simulink model "ACC_CC_model_best_2017aV1"  (Simulink 9.0)
settings: Solver=FixedStepAuto  StartTime=0.0  StopTime=1000  RelTol=1e-3
InitFcn:
  | step=0.001;%时间步长
  | run par.m
values from neighbouring files (symbols this model uses):
  ax_1 = Pop(i,1)    [IGPSO.m]
  ax_2 = Pop(i,2)    [IGPSO.m]
  ess_init_soc = 0.9    [IGPSO.m]
  ess_max_ah_cap = 5    [IGPSO.m]
  ess_r_chg = [0.001393 0.001393 0.001393 0.001393 0.001256 0.001172 0.001099 0.001074 0.001058 0.001066 0.0011 0.001161 0.001244 0.001327 0.001327]*3/5*32    [IGPSO.m]
  ess_r_dis = [0.004178 0.004178 0.004178 0.004178 0.003769 0.003517 0.003296 0.003222 0.003173 0.003197 0.0033 0.003483 0.003732 0.00398 0.00398]*3/5*32    [IGPSO.m]
  ess_soc = [0 0.2 0.25 0.3 0.35 0.4 0.45 0.5 0.55 0.6 0.65 0.7 0.75 0.8 1]    [IGPSO.m]
  ess_voc = [3.124 3.36 3.42 3.479 3.501 3.524 3.547 3.569 3.593 3.616 3.65 3.684 3.72 3.756 3.9]*3*32    [IGPSO.m]
  mc_eff_map = [0.43,0.49,0.58,0.66,0.73,0.70,0.73,0.66,0.58,0.49,0.43 ... (first row only)    [IGPSO.m]
  mc_map_spd = [0;1000;2000;3000;3500;4000;5000;6000;6500;7000;8000]*(2*pi)/60    [IGPSO.m]
  mc_map_trq = motorMAP(1,2:end)    [IGPSO.m]
  mc_max_trq = [142.2;148.6;146.5;92.4;83.9;71.1;56.9;48.4;43.4;37.7;35.6]    [IGPSO.m]
  v_base = 30    [IGPSO.m]
libraries: simulink x2, Solver_SF x1
(part 1 of 2)
settings Model: Creator=Administrator  LastModifiedBy=61602
settings DataIOCC: SaveFormat=Dataset
settings OptimizationCC: LifeSpan=auto
settings DebuggingCC: UnderspecifiedInitializationDetection=Simplified  MergeDetectMultiDrivingBlocksExec=error  SFUnexpectedBacktrackingDiag=error  SFNoUnconditionalDefaultTransitionDiag=error  SFExecutionAtInitializationDiag=warning
settings HardwareCC: ProdBitPerPointer=64  ProdBitPerSizeT=64  ProdBitPerPtrDiffT=64  ProdLargestAtomicFloat=Float  ProdIntDivRoundTo=Zero  ProdEndianess=LittleEndian  ProdWordSize=64  ProdHWDeviceType=Intel->x86-64 (Windows64)
settings ModelReferenceCC: PropagateSignalLabelsOutOfModel=on
settings GRTTargetCC: TargetLangStandard=C99 (ISO)
settings ConfigComp: CovMetricSettings=dwe  CovHtmlReporting=off  CovSaveCumulativeToWorkspaceVar=off  CovSaveSingleToWorkspaceVar=off  CovExternalEMLEnable=on

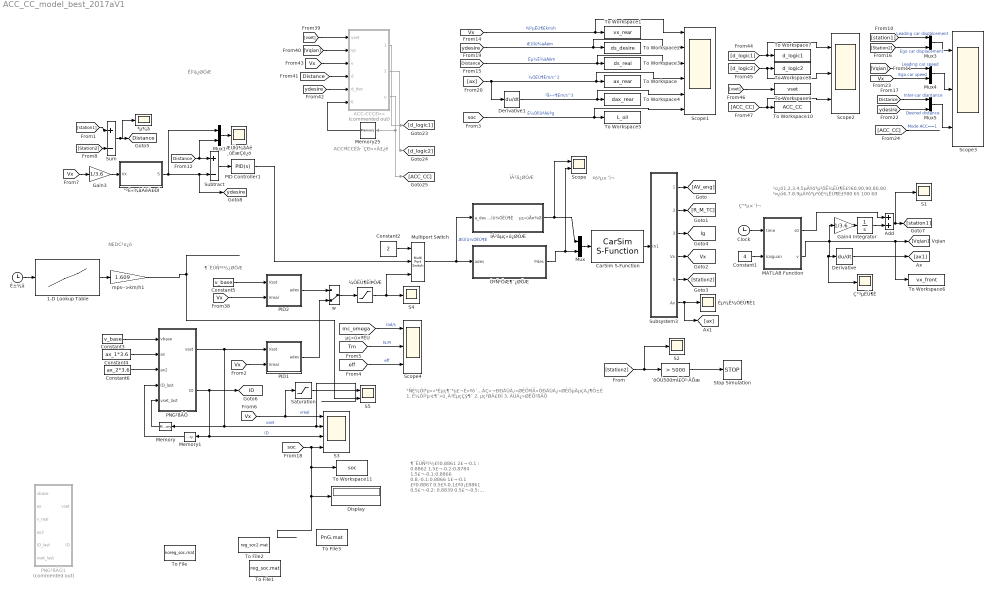
== system ACC_CC_model_best_2017aV1 ==
  note: NEDC工况
  note: 把燃油车换成电动车，然后搭建电池模型，能量回收策略模型png滑行最优加速度用粒子群或者遗传算法优化去做，最后对比考虑滑行能量回收和没有能量回收的电量对比
      | 1. 燃油车发动机改成电驱动
      | 2. 电池模型
      | 3. 能量回收策略
  note: ACC和CC算法切换模块
  note: 工况1,2,3,4,5的后车初始速度：60,90,90,80,80
      | 工况6.7.8.9的后车初始速度：80   65 100 60
  note: 下层控制
  note: 定速巡航控制
  note: 前车状态
  note: 后车状态
  note: 上层控制
  note: 定速巡航：0.8861
      | 2，-0.1 :  0.8862
      | 1.5，-0.2:0.8784
      | 1.5，-0.1:0.8866
      | 0.8,-0.1:0.8866
      | 1，-0.1 ：0.8867
      | 0.5：-0.1：0。8861
      | 0.5，-0.2: 0.8839
      | 0.5，-0.5: 0.8801
      | 0.5，-1； 0.8796
      | 0.5，-2:   0.8721
  1-D Lookup Table : Lookup_n-D  NumberOfTableDimensions=1  BreakpointsForDimension1=0:1179  Table=|  ExtrapMethod=Clip  UseLastTableValue=on  InternalRulePriority=Speed  RndMeth=Simplest  InputSameDT=on
      | [0
      | 0
      | 0
      | 0
      | 0
      | 0
      | 0
      | 0
      | 0
      | 0
      | 0
      | 2.36120600000000
      | 4.66027500000000
      | 7.02148100000000
      | 9.32055000000000
      | 9.32055000000000
      | 9.32055000000000
      | 9.32055000000000
      | 9.32055000000000
      | 9.32055000000000
      | 9.32055000000000
      | 9.32055000000000
      | 9.32055000000000
      | 7.45644000000000
      | 5.59233000000000
      | 3.72822000000000
      | 1.86411000000000
      | 0
      | 0
      | 0
      | 0
      | 0
      | 0
      | 0
      | 0
      | 0
      | 0
      | 0
      | 0
      | 0
      | 0
      | 0
      | 0
      | 0
      | 0
      | 0
      | 0
      | 0
      | 0
      | 1.67769900000000
      | 3.29326100000000
      | 4.97096000000000
      | 6.64865900000000
      | 8.26422100000000
      | 9.94192000000000
      | 11.6196190000000
      | 13.2351810000000
      | 14.9128800000000
      | 16.5905790000000
      | 18.2061410000000
      | 19.8838400000000
      | 19.8838400000000
      | 19.8838400000000
      | 19.8838400000000
      | 19.8838400000000
      | 19.8838400000000
      | 19.8838400000000
      | 19.8838400000000
      | 19.8838400000000
      | 19.8838400000000
      | 19.8838400000000
      | 19.8838400000000
      | 19.8838400000000
      | 19.8838400000000
      | 19.8838400000000
      | 19.8838400000000
      | 19.8838400000000
      | 19.8838400000000
      | 19.8838400000000
      | 19.8838400000000
      | 19.8838400000000
      | 19.8838400000000
      | 19.8838400000000
      | 19.8838400000000
      | 19.8838400000000
      | 18.0818670000000
      | 16.2798940000000
      | 14.4779210000000
      | 12.6759480000000
      | 10.8739750000000
      | 9.00986500000000
      | 7.20789200000000
      | 5.40591900000000
      | 3.60394600000000
      | 1.80197300000000
      | 0
      | 0
      | 0
      | 0
      | 0
      | 0
      | 0
      | 0
      | 0
      | 0
      | 0
      | 0
      | 0
      | 0
      | 0
      | 0
      | 0
      | 0
      | 0
      | 0
      | 0
      | 0
      | 1.18060300000000
      | 2.36120600000000
      | 3.60394600000000
      | 4.78454900000000
      | 5.96515200000000
      | 7.14575500000000
      | 8.38849500000000
      | 9.56909800000000
      | 10.7497010000000
      | 11.9303040000000
      | 13.1730440000000
      | 14.5400580000000
      | 15.5342500000000
      | 16.7148530000000
      | 17.8954560000000
      | 19.1381960000000
      | 20.3187990000000
      | 21.4994020000000
      | 22.6800050000000
      | 23.9227450000000
      | 25.1033480000000
      | 26.2839510000000
      | 27.4645540000000
      | 28.7072940000000
      | 29.8878970000000
      | 31.0685000000000
      | 31.0685000000000
      | 31.0685000000000
      | 31.0685000000000
      | 31.0685000000000
      | 31.0685000000000
      | 31.0685000000000
      | 31.0685000000000
      | 31.0685000000000
      | 31.0685000000000
      | 31.0685000000000
      | 31.0685000000000
      | 31.0685000000000
      | 29.8878970000000
      | 28.7072940000000
      | 27.5888280000000
      | 26.4082250000000
      | 25.2276220000000
      | 24.1091560000000
      | 22.9285530000000
      | 21.7479500000000
      | 21.7479500000000
      | 21.7479500000000
      | 21.7479500000000
      | 21.7479500000000
      | 21.7479500000000
      | 21.7479500000000
      | 21.7479500000000
      | 21.7479500000000
      | 21.7479500000000
      | 21.7479500000000
      | 21.7479500000000
      | 21.7479500000000
      | 21.7479500000000
      | 19.9459770000000
      | 18.1440040000000
      | 16.2798940000000
      | 14.4779210000000
      | 12.6759480000000
      | 10.8739750000000
      | 9.07200200000000
      | 7.27002900000000
      | 5.40591900000000
      | 3.60394600000000
      | 1.80197300000000
      | 0
      | 0
      | 0
      | 0
      | 0
      | 0
      | 0
      | 0
      | 0
      | 0
      | 0
      | 0
      | 0
      | 0
      | 0
      | 0
      | 0
      | 0
      | 0
      | 2.36120600000000
      | 4.66027500000000
      | 7.02148100000000
      | 9.32055000000000
      | 9.32055000000000
      | 9.32055000000000
      | 9.32055000000000
      | 9.32055000000000
      | 9.32055000000000
      | 9.32055000000000
      | 9.32055000000000
      | 9.32055000000000
      | 7.45644000000000
      | 5.59233000000000
      | 3.72822000000000
      | 1.86411000000000
      | 0
      | 0
      | 0
      | 0
      | 0
      | 0
      | 0
      | 0
      | 0
      | 0
      | 0
      | 0
      | 0
      | 0
      | 0
      | 0
      | 0
      | 0
      | 0
      | 0
      | 0
      | 0
      | 1.67769900000000
      | 3.29326100000000
      | 4.97096000000000
      | 6.64865900000000
      | 8.26422100000000
      | 9.94192000000000
      | 11.6196190000000
      | 13.2351810000000
      | 14.9128800000000
      | 16.5905790000000
      | 18.2061410000000
      | 19.8838400000000
      | 19.8838400000000
      | 19.8838400000000
      | 19.8838400000000
      | 19.8838400000000
      | 19.8838400000000
      | 19.8838400000000
      | 19.8838400000000
      | 19.8838400000000
      | 19.8838400000000
      | 19.8838400000000
      | 19.8838400000000
      | 19.8838400000000
      | 19.8838400000000
      | 19.8838400000000
      | 19.8838400000000
      | 19.8838400000000
      | 19.8838400000000
      | 19.8838400000000
      | 19.8838400000000
      | 19.8838400000000
      | 19.8838400000000
      | 19.8838400000000
      | 19.8838400000000
      | 19.8838400000000
      | 18.0818670000000
      | 16.2798940000000
      | 14.4779210000000
      | 12.6759480000000
      | 10.8739750000000
      | 9.00986500000000
      | 7.20789200000000
      | 5.40591900000000
      | 3.60394600000000
      | 1.80197300000000
      | 0
      | 0
      | 0
      | 0
      | 0
      | 0
      | 0
      | 0
      | 0
      | 0
      | 0
      | 0
      | 0
      | 0
      | 0
      | 0
      | 0
      | 0
      | 0
      | 0
      | 0
      | 0
      | 1.18060300000000
      | 2.36120600000000
      | 3.60394600000000
      | 4.78454900000000
      | 5.96515200000000
      | 7.14575500000000
      | 8.38849500000000
      | 9.56909800000000
      | 10.7497010000000
      | 11.9303040000000
      | 13.1730440000000
      | 14.5400580000000
      | 15.5342500000000
      | 16.7148530000000
      | 17.8954560000000
      | 19.1381960000000
      | 20.3187990000000
      | 21.4994020000000
      | 22.6800050000000
      | 23.9227450000000
      | 25.1033480000000
      | 26.2839510000000
      | 27.4645540000000
      | 28.7072940000000
      | 29.8878970000000
      | 31.0685000000000
      | 31.0685000000000
      | 31.0685000000000
      | 31.0685000000000
      | 31.0685000000000
      | 31.0685000000000
      | 31.0685000000000
      | 31.0685000000000
      | 31.0685000000000
      | 31.0685000000000
      | 31.0685000000000
      | 31.0685000000000
      | 31.0685000000000
      | 29.8878970000000
      | 28.7072940000000
      | 27.5888280000000
      | 26.4082250000000
      | 25.2276220000000
      | 24.1091560000000
      | 22.9285530000000
      | 21.7479500000000
      | 21.7479500000000
      | 21.7479500000000
      | 21.7479500000000
      | 21.7479500000000
      | 21.7479500000000
      | 21.7479500000000
      | 21.7479500000000
      | 21.7479500000000
      | 21.7479500000000
      | 21.7479500000000
      | 21.7479500000000
      | 21.7479500000000
      | 21.7479500000000
      | 19.9459770000000
      | 18.1440040000000
      | 16.2798940000000
      | 14.4779210000000
      | 12.6759480000000
      | 10.8739750000000
      | 9.07200200000000
      | 7.27002900000000
      | 5.40591900000000
      | 3.60394600000000
      | 1.80197300000000
      | 0
      | 0
      | 0
      | 0
      | 0
      | 0
      | 0
      | 0
      | 0
      | 0
      | 0
      | 0
      | 0
      | 0
      | 0
      | 0
      | 0
      | 0
      | 0
      | 2.36120600000000
      | 4.66027500000000
      | 7.02148100000000
      | 9.32055000000000
      | 9.32055000000000
      | 9.32055000000000
      | 9.32055000000000
      | 9.32055000000000
      | 9.32055000000000
      | 9.32055000000000
      | 9.32055000000000
      | 9.32055000000000
      | 7.45644000000000
      | 5.59233000000000
      | 3.72822000000000
      | 1.86411000000000
      | 0
      | 0
      | 0
      | 0
      | 0
      | 0
      | 0
      | 0
      | 0
      | 0
      | 0
      | 0
      | 0
      | 0
      | 0
      | 0
      | 0
      | 0
      | 0
      | 0
      | 0
      | 0
      | 1.67769900000000
      | 3.29326100000000
      | 4.97096000000000
      | 6.64865900000000
      | 8.26422100000000
      | 9.94192000000000
      | 11.6196190000000
      | 13.2351810000000
      | 14.9128800000000
      | 16.5905790000000
      | 18.2061410000000
      | 19.8838400000000
      | 19.8838400000000
      | 19.8838400000000
      | 19.8838400000000
      | 19.8838400000000
      | 19.8838400000000
      | 19.8838400000000
      | 19.8838400000000
      | 19.8838400000000
      | 19.8838400000000
      | 19.8838400000000
      | 19.8838400000000
      | 19.8838400000000
      | 19.8838400000000
      | 19.8838400000000
      | 19.8838400000000
      | 19.8838400000000
      | 19.8838400000000
      | 19.8838400000000
      | 19.8838400000000
      | 19.8838400000000
      | 19.8838400000000
      | 19.8838400000000
      | 19.8838400000000
      | 19.8838400000000
      | 18.0818670000000
      | 16.2798940000000
      | 14.4779210000000
      | 12.6759480000000
      | 10.8739750000000
      | 9.00986500000000
      | 7.20789200000000
      | 5.40591900000000
      | 3.60394600000000
      | 1.80197300000000
      | 0
      | 0
      | 0
      | 0
      | 0
      | 0
      | 0
      | 0
      | 0
      | 0
      | 0
      | 0
      | 0
      | 0
      | 0
      | 0
      | 0
      | 0
      | 0
      | 0
      | 0
      | 0
      | 1.18060300000000
      | 2.36120600000000
      | 3.60394600000000
      | 4.78454900000000
      | 5.96515200000000
      | 7.14575500000000
      | 8.38849500000000
      | 9.56909800000000
      | 10.7497010000000
      | 11.9303040000000
      | 13.1730440000000
      | 14.5400580000000
      | 15.5342500000000
      | 16.7148530000000
      | 17.8954560000000
      | 19.1381960000000
      | 20.3187990000000
      | 21.4994020000000
      | 22.6800050000000
      | 23.9227450000000
      | 25.1033480000000
      | 26.2839510000000
      | 27.4645540000000
      | 28.7072940000000
      | 29.8878970000000
      | 31.0685000000000
      | 31.0685000000000
      | 31.0685000000000
      | 31.0685000000000
      | 31.0685000000000
      | 31.0685000000000
      | 31.0685000000000
      | 31.0685000000000
      | 31.0685000000000
      | 31.0685000000000
      | 31.0685000000000
      | 31.0685000000000
      | 31.0685000000000
      | 29.8878970000000
      | 28.7072940000000
      | 27.5888280000000
      | 26.4082250000000
      | 25.2276220000000
      | 24.1091560000000
      | 22.9285530000000
      | 21.7479500000000
      | 21.7479500000000
      | 21.7479500000000
      | 21.7479500000000
      | 21.7479500000000
      | 21.7479500000000
      | 21.7479500000000
      | 21.7479500000000
      | 21.7479500000000
      | 21.7479500000000
      | 21.7479500000000
      | 21.7479500000000
      | 21.7479500000000
      | 21.7479500000000
      | 19.9459770000000
      | 18.1440040000000
      | 16.2798940000000
      | 14.4779210000000
      | 12.6759480000000
      | 10.8739750000000
      | 9.07200200000000
      | 7.27002900000000
      | 5.40591900000000
      | 3.60394600000000
      | 1.80197300000000
      | 0
      | 0
      | 0
      | 0
      | 0
      | 0
      | 0
      | 0
      | 0
      | 0
      | 0
      | 0
      | 0
      | 0
      | 0
      | 0
      | 0
      | 0
      | 0
      | 2.36120600000000
      | 4.66027500000000
      | 7.02148100000000
      | 9.32055000000000
      | 9.32055000000000
      | 9.32055000000000
      | 9.32055000000000
      | 9.32055000000000
      | 9.32055000000000
      | 9.32055000000000
      | 9.32055000000000
      | 9.32055000000000
      | 7.45644000000000
      | 5.59233000000000
      | 3.72822000000000
      | 1.86411000000000
      | 0
      | 0
      | 0
      | 0
      | 0
      | 0
      | 0
      | 0
      | 0
      | 0
      | 0
      | 0
      | 0
      | 0
      | 0
      | 0
      | 0
      | 0
      | 0
      | 0
      | 0
      | 0
      | 1.67769900000000
      | 3.29326100000000
      | 4.97096000000000
      | 6.64865900000000
      | 8.26422100000000
      | 9.94192000000000
      | 11.6196190000000
      | 13.2351810000000
      | 14.9128800000000
      | 16.5905790000000
      | 18.2061410000000
      | 19.8838400000000
      | 19.8838400000000
      | 19.8838400000000
      | 19.8838400000000
      | 19.8838400000000
      | 19.8838400000000
      | 19.8838400000000
      | 19.8838400000000
      | 19.8838400000000
      | 19.8838400000000
      | 19.8838400000000
      | 19.8838400000000
      | 19.8838400000000
      | 19.8838400000000
      | 19.8838400000000
      | 19.8838400000000
      | 19.8838400000000
      | 19.8838400000000
      | 19.8838400000000
      | 19.8838400000000
      | 19.8838400000000
      | 19.8838400000000
      | 19.8838400000000
      | 19.8838400000000
      | 19.8838400000000
      | 18.0818670000000
      | 16.2798940000000
      | 14.4779210000000
      | 12.6759480000000
      | 10.8739750000000
      | 9.00986500000000
      | 7.20789200000000
      | 5.40591900000000
      | 3.60394600000000
      | 1.80197300000000
      | 0
      | 0
      | 0
      | 0
      | 0
      | 0
      | 0
      | 0
      | 0
      | 0
      | 0
      | 0
      | 0
      | 0
      | 0
      | 0
      | 0
      | 0
      | 0
      | 0
      | 0
      | 0
      | 1.18060300000000
      | 2.36120600000000
      | 3.60394600000000
      | 4.78454900000000
      | 5.96515200000000
      | 7.14575500000000
      | 8.38849500000000
      | 9.56909800000000
      | 10.7497010000000
      | 11.9303040000000
      | 13.1730440000000
      | 14.5400580000000
      | 15.5342500000000
      | 16.7148530000000
      | 17.8954560000000
      | 19.1381960000000
      | 20.3187990000000
      | 21.4994020000000
      | 22.6800050000000
      | 23.9227450000000
      | 25.1033480000000
      | 26.2839510000000
      | 27.4645540000000
      | 28.7072940000000
      | 29.8878970000000
      | 31.0685000000000
      | 31.0685000000000
      | 31.0685000000000
      | 31.0685000000000
      | 31.0685000000000
      | 31.0685000000000
      | 31.0685000000000
      | 31.0685000000000
      | 31.0685000000000
      | 31.0685000000000
      | 31.0685000000000
      | 31.0685000000000
      | 31.0685000000000
      | 29.8878970000000
      | 28.7072940000000
      | 27.5888280000000
      | 26.4082250000000
      | 25.2276220000000
      | 24.1091560000000
      | 22.9285530000000
      | 21.7479500000000
      | 21.7479500000000
      | 21.7479500000000
      | 21.7479500000000
      | 21.7479500000000
      | 21.7479500000000
      | 21.7479500000000
      | 21.7479500000000
      | 21.7479500000000
      | 21.7479500000000
      | 21.7479500000000
      | 21.7479500000000
      | 21.7479500000000
      | 21.7479500000000
      | 19.9459770000000
      | 18.1440040000000
      | 16.2798940000000
      | 14.4779210000000
      | 12.6759480000000
      | 10.8739750000000
      | 9.07200200000000
      | 7.27002900000000
      | 5.40591900000000
      | 3.60394600000000
      | 1.80197300000000
      | 0
      | 0
      | 0
      | 0
      | 0
      | 0
      | 0
      | 0
      | 0
      | 0
      | 0
      | 0
      | 0
      | 0
      | 0
      | 0
      | 0
      | 0
      | 0
      | 0
      | 0
      | 0
      | 0
      | 0
      | 0
      | 0
      | 0
      | 0
      | 1.86411000000000
      | 3.72822000000000
      | 5.59233000000000
      | 7.45644000000000
      | 9.32055000000000
      | 9.32055000000000
      | 9.32055000000000
      | 10.6875640000000
      | 12.0545780000000
      | 13.4837290000000
      | 14.8507430000000
      | 16.2177570000000
      | 17.5847710000000
      | 19.0139220000000
      | 20.3809360000000
      | 21.7479500000000
      | 21.7479500000000
      | 21.7479500000000
      | 22.9285530000000
      | 24.1091560000000
      | 25.2276220000000
      | 26.4082250000000
      | 27.5888280000000
      | 28.7694310000000
      | 29.8878970000000
      | 31.0685000000000
      | 31.0685000000000
      | 31.0685000000000
      | 32.0005550000000
      | 32.9947470000000
      | 33.9268020000000
      | 34.9209940000000
      | 35.8530490000000
      | 36.7851040000000
      | 37.7792960000000
      | 38.7113510000000
      | 39.6434060000000
      | 40.6375980000000
      | 41.5696530000000
      | 42.5638450000000
      | 43.4959000000000
      | 43.4959000000000
      | 43.4959000000000
      | 43.4959000000000
      | 43.4959000000000
      | 43.4959000000000
      | 43.4959000000000
      | 43.4959000000000
      | 43.4959000000000
      | 43.4959000000000
      | 43.4959000000000
      | 43.4959000000000
      | 43.4959000000000
      | 43.4959000000000
      | 43.4959000000000
      | 43.4959000000000
      | 43.4959000000000
      | 43.4959000000000
      | 43.4959000000000
      | 43.4959000000000
      | 43.4959000000000
      | 43.4959000000000
      | 43.4959000000000
      | 43.4959000000000
      | 43.4959000000000
      | 43.4959000000000
      | 43.4959000000000
      | 43.4959000000000
      | 43.4959000000000
      | 43.4959000000000
      | 43.4959000000000
      | 43.4959000000000
      | 43.4959000000000
      | 43.4959000000000
      | 43.4959000000000
      | 43.4959000000000
      | 43.4959000000000
      | 43.4959000000000
      | 43.4959000000000
      | 43.4959000000000
      | 43.4959000000000
      | 43.4959000000000
      | 43.4959000000000
      | 43.4959000000000
      | 43.4959000000000
      | 43.4959000000000
      | 43.4959000000000
      | 43.4959000000000
      | 43.4959000000000
      | 43.4959000000000
      | 43.4959000000000
      | 41.9424750000000
      | 40.3890500000000
      | 38.8356250000000
      | 37.2822000000000
      | 35.7287750000000
      | 34.1753500000000
      | 32.6219250000000
      | 31.0685000000000
      | 31.0685000000000
      | 31.0685000000000
      | 31.0685000000000
      | 31.0685000000000
      | 31.0685000000000
      | 31.0685000000000
      | 31.0685000000000
      | 31.0685000000000
      | 31.0685000000000
      | 31.0685000000000
      | 31.0685000000000
      | 31.0685000000000
      | 31.0685000000000
      | 31.0685000000000
      | 31.0685000000000
      | 31.0685000000000
      | 31.0685000000000
      | 31.0685000000000
      | 31.0685000000000
      | 31.0685000000000
      | 31.0685000000000
      | 31.0685000000000
      | 31.0685000000000
      | 31.0685000000000
      | 31.0685000000000
      | 31.0685000000000
      | 31.0685000000000
      | 31.0685000000000
      | 31.0685000000000
      | 31.0685000000000
      | 31.0685000000000
      | 31.0685000000000
      | 31.0685000000000
      | 31.0685000000000
      | 31.0685000000000
      | 31.0685000000000
      | 31.0685000000000
      | 31.0685000000000
      | 31.0685000000000
      | 31.0685000000000
      | 31.0685000000000
      | 31.0685000000000
      | 31.0685000000000
      | 31.0685000000000
      | 31.0685000000000
      | 31.0685000000000
      | 31.0685000000000
      | 31.0685000000000
      | 31.0685000000000
      | 31.0685000000000
      | 31.0685000000000
      | 31.0685000000000
      | 31.0685000000000
      | 31.0685000000000
      | 31.0685000000000
      | 31.0685000000000
      | 31.0685000000000
      | 31.0685000000000
      | 31.0685000000000
      | 31.0685000000000
      | 31.0685000000000
      | 31.0685000000000
      | 31.0685000000000
      | 31.0685000000000
      | 31.0685000000000
      | 31.0685000000000
      | 31.0685000000000
      | 31.0685000000000
      | 31.0685000000000
      | 32.0005550000000
      | 32.9947470000000
      | 33.9268020000000
      | 34.9209940000000
      | 35.8530490000000
      | 36.7851040000000
      | 37.7792960000000
      | 38.7113510000000
      | 39.6434060000000
      | 40.6375980000000
      | 41.5696530000000
      | 42.5638450000000
      | 43.4959000000000
      | 43.4959000000000
      | 43.4959000000000
      | 43.4959000000000
      | 43.4959000000000
      | 43.4959000000000
      | 43.4959000000000
      | 43.4959000000000
      | 43.4959000000000
      | 43.4959000000000
      | 43.4959000000000
      | 43.4959000000000
      | 43.4959000000000
      | 43.4959000000000
      | 43.4959000000000
      | 43.4959000000000
      | 43.4959000000000
      | 43.4959000000000
      | 43.4959000000000
      | 43.4959000000000
      | 43.4959000000000
      | 43.4959000000000
      | 43.4959000000000
      | 43.4959000000000
      | 43.4959000000000
      | 43.4959000000000
      | 43.4959000000000
      | 43.4959000000000
      | 43.4959000000000
      | 43.4959000000000
      | 43.4959000000000
      | 43.4959000000000
      | 43.4959000000000
      | 43.4959000000000
      | 43.4959000000000
      | 43.4959000000000
      | 43.4959000000000
      | 43.4959000000000
      | 43.4959000000000
      | 43.4959000000000
      | 43.4959000000000
      | 43.4959000000000
      | 43.4959000000000
      | 43.4959000000000
      | 43.4959000000000
      | 43.4959000000000
      | 43.4959000000000
      | 43.4959000000000
      | 43.4959000000000
      | 43.4959000000000
      | 43.4959000000000
      | 44.0551330000000
      | 44.5522290000000
      | 45.1114620000000
      | 45.6085580000000
      | 46.1677910000000
      | 46.6648870000000
      | 47.2241200000000
      | 47.7833530000000
      | 48.2804490000000
      | 48.8396820000000
      | 49.3367780000000
      | 49.8960110000000
      | 50.3931070000000
      | 50.9523400000000
      | 51.5115730000000
      | 52.0086690000000
      | 52.5679020000000
      | 53.0649980000000
      | 53.6242310000000
      | 54.1213270000000
      | 54.6805600000000
      | 55.2397930000000
      | 55.7368890000000
      | 56.2961220000000
      | 56.7932180000000
      | 57.3524510000000
      | 57.8495470000000
      | 58.4087800000000
      | 58.9680130000000
      | 59.4651090000000
      | 60.0243420000000
      | 60.5214380000000
      | 61.0806710000000
      | 61.5777670000000
      | 62.1370000000000
      | 62.1370000000000
      | 62.1370000000000
      | 62.1370000000000
      | 62.1370000000000
      | 62.1370000000000
      | 62.1370000000000
      | 62.1370000000000
      | 62.1370000000000
      | 62.1370000000000
      | 62.1370000000000
      | 62.1370000000000
      | 62.1370000000000
      | 62.1370000000000
      | 62.1370000000000
      | 62.1370000000000
      | 62.1370000000000
      | 62.1370000000000
      | 62.1370000000000
      | 62.1370000000000
      | 62.1370000000000
      | 62.1370000000000
      | 62.1370000000000
      | 62.1370000000000
      | 62.1370000000000
      | 62.1370000000000
      | 62.1370000000000
      | 62.1370000000000
      | 62.1370000000000
      | 62.1370000000000
      | 62.1370000000000
      | 62.7583700000000
      | 63.3797400000000
      | 64.0011100000000
      | 64.6224800000000
      | 65.2438500000000
      | 65.8652200000000
      | 66.4865900000000
      | 67.1079600000000
      | 67.7293300000000
      | 68.3507000000000
      | 68.9720700000000
      | 69.5934400000000
      | 70.2148100000000
      | 70.8361800000000
      | 71.4575500000000
      | 72.0789200000000
      | 72.7002900000000
      | 73.3216600000000
      | 73.9430300000000
      | 74.5644000000000
      | 74.5644000000000
      | 74.5644000000000
      | 74.5644000000000
      | 74.5644000000000
      | 74.5644000000000
      | 74.5644000000000
      | 74.5644000000000
      | 74.5644000000000
      | 74.5644000000000
      | 74.5644000000000
      | 73.0109750000000
      | 71.4575500000000
      | 69.9041250000000
      | 68.3507000000000
      | 66.7972750000000
      | 65.2438500000000
      | 63.6904250000000
      | 62.1370000000000
      | 60.5835750000000
      | 59.0301500000000
      | 57.4767250000000
      | 55.9233000000000
      | 54.3698750000000
      | 52.8164500000000
      | 51.2630250000000
      | 49.7096000000000
      | 47.4105310000000
      | 45.0493250000000
      | 42.7502560000000
      | 40.3890500000000
      | 38.0899810000000
      | 35.7287750000000
      | 33.4297060000000
      | 31.0685000000000
      | 27.9616500000000
      | 24.8548000000000
      | 21.7479500000000
      | 18.6411000000000
      | 15.5342500000000
      | 12.4274000000000
      | 9.32055000000000
      | 6.21370000000000
      | 3.10685000000000
      | 0
      | 0
      | 0
      | 0
      | 0
      | 0
      | 0
      | 0
      | 0
      | 0
      | 0
      | 0
      | 0
      | 0
      | 0
      | 0
      | 0
      | 0
      | 0
      | 0
      | 0]
  ACC-CC切换 : MATLAB Function  Commented=on  TreatAsAtomicUnit=on
  Add : Sum
  CarSim S-Function : Solver_SF/CarSim S-Function  Priority=1  VehicleCode=i_i2  SIMFILE=simfile.sim
  Clock : Clock
  Constant1 : Constant  Value=4
  Constant2 : Constant  Value=2
  Constant3 : Constant  Value=v_base
  Constant4 : Constant  Value=ax_1*3.6
  Constant5 : Constant  Value=v_base
  Constant6 : Constant  Value=ax_2*3.6
  Derivative : Derivative
  Derivative1 : Derivative
  Display : Display
  Gain3 : Gain  Gain=1/3.6
  Gain4 : Gain  Gain=1/3.6
  Integrator : Integrator
  MATLAB Function : MATLAB Function  TreatAsAtomicUnit=on
  Memory : Memory  InitialCondition=v_base
  Memory1 : Memory  InitialCondition=1
  Memory25 : Memory
  Multiport Switch : MultiPortSwitch  Inputs=2
  Mux{,1,3..5} (5 alike) : Mux  Inputs=2
  PID Controller1 : simulink/Continuous/PID Controller  Controller=PID  TimeDomain=Continuous-time  SampleTime=-1  IntegratorMethod=Forward Euler  FilterMethod=Forward Euler  Form=Parallel  UseFilter=on  ControllerParametersSource=internal  P=4  I=0.01  D=2  N=100  InitialConditionSource=internal  InitialConditionForIntegrator=0  InitialConditionForFilter=0  ExternalReset=none  LimitOutput=off  UpperSaturationLimit=inf  LowerSaturationLimit=-inf  LinearizeAsGain=on  AntiWindupMode=none  Kb=1  TrackingMode=off  Kt=1  PParamMin=[]  PParamMax=[]  IParamMin=[]  IParamMax=[]  DParamMin=[]  DParamMax=[]  NParamMin=[]  NParamMax=[]  KbParamMin=[]  KbParamMax=[]  KtParamMin=[]  KtParamMax=[]  POutMin=[]  POutMax=[]  IOutMin=[]  IOutMax=[]  DOutMin=[]  DOutMax=[]  NOutMin=[]  NOutMax=[]  KbOutMin=[]  KbOutMax=[]  KtOutMin=[]  KtOutMax=[]  IntegratorOutMin=[]  IntegratorOutMax=[]  FilterOutMin=[]  FilterOutMax=[]  SumOutMin=[]  SumOutMax=[]  SumI1OutMin=[]  SumI1OutMax=[]  SumI2OutMin=[]  SumI2OutMax=[]  SumI3OutMin=[]  SumI3OutMax=[]  SumDOutMin=[]  SumDOutMax=[]  SaturationOutMin=[]  SaturationOutMax=[]  IntegratorContinuousStateAttributes=''  IntegratorStateMustResolveToSignalObject=off  IntegratorRTWStateStorageClass=Auto  FilterContinuousStateAttributes=''  FilterStateMustResolveToSignalObject=off  FilterRTWStateStorageClass=Auto  DifferentiatorICPrevScaledInput=0  DifferentiatorOutMin=[]  DifferentiatorOutMax=[]  FilterDiffOutCoefMin=[]  FilterDiffOutCoefMax=[]  SumDenOutMin=[]  SumDenOutMax=[]  SumNumOutMin=[]  SumNumOutMax=[]  ReciprocalOutMin=[]  ReciprocalOutMax=[]  DivideOutMin=[]  DivideOutMax=[]  TunerSelectOption=Transfer Function Based (PID Tuner App)
  PID1 : Subsystem
  PID2 : Subsystem
  PNG策略 : MATLAB Function  TreatAsAtomicUnit=on
  PNG策略1 : MATLAB Function  Commented=on  TreatAsAtomicUnit=on
  S1 : Scope
  S2 : Scope
  S3 : Scope  NumInputPorts=4
  S4 : Scope
  S5 : Scope  NumInputPorts=2
  Saturation : Saturate  UpperLimit=1111000  LowerLimit=0
  Scope : Scope  NumInputPorts=2
  Scope1 : Scope  NumInputPorts=6
  Scope2 : Scope  NumInputPorts=3
  Scope3 : Scope  NumInputPorts=3
  Scope4 : Scope  NumInputPorts=3
  Stop Simulation : Stop
  Subsystem3 : Subsystem
  Subtract : Sum  Inputs=+-
  Sum : Sum  Inputs=+|-
  To File : ToFile  Filename=noreg_soc.mat  MatrixName=ans2  SaveFormat=Timeseries
  To File1 : ToFile  Filename=reg_soc.mat  SaveFormat=Timeseries
  To File2 : ToFile  Filename=reg_soc2.mat  MatrixName=ans4  SaveFormat=Timeseries
  To File3 : ToFile  Filename=PnG.mat  MatrixName=ans6  SaveFormat=Timeseries
  To Workspace : ToWorkspace  VariableName=ax_rear  SampleTime=-1
  To Workspace1 : ToWorkspace  VariableName=vx_rear  SampleTime=-1
  To Workspace10 : ToWorkspace  VariableName=ACC_CC  SampleTime=-1
  To Workspace11 : ToWorkspace  VariableName=soc  SampleTime=-1
  To Workspace2 : ToWorkspace  VariableName=ds_desire  SampleTime=-1
  To Workspace3 : ToWorkspace  VariableName=ds_real  SampleTime=-1
  To Workspace4 : ToWorkspace  VariableName=dax_rear  SampleTime=-1
  To Workspace5 : ToWorkspace  VariableName=L_oil  SampleTime=-1
  To Workspace6 : ToWorkspace  VariableName=vx_front  SampleTime=-1
  To Workspace7 : ToWorkspace  VariableName=d_logic1  SampleTime=-1
  To Workspace8 : ToWorkspace  VariableName=d_logic2  SampleTime=-1
  To Workspace9 : ToWorkspace  VariableName=vset  SampleTime=-1
  mps-->km/h1 : Gain  Gain=1.609
  w : ManualSwitch  CurrentSetting=0
  下层电机控制 : Subsystem
  前车速度 : Scope
  加速度限制 : Saturate  UpperLimit=9  LowerLimit=-9
  大于500m停止仿真 : simulink/Logic and Bit Operations/Compare To Constant  relop=>  const=5000  OutDataTypeStr=boolean
  安全距离模型 : Subsystem
  实际加速度1 : Scope
  时间 : Clock
  期望距离 跟随情况 : Scope
  液压制动控制 : Subsystem
  车距 : Scope
  tag scope: Distance=global, ID=global, Ig=global, Vx=global, ydesire=global
  wires:
  Subtract/1 -> PID Controller1/1
  安全距离模型/1(S) -> Subtract/2, [ydesire], Mux1/1
  液压制动控制/1("Pdes ") -> Mux/2, Scope/2
  CarSim S-Function/1 -> Subsystem3/1(In1)
  Mux/1 -> CarSim S-Function/1
  Subsystem3/6(Ax) -> [ax], 实际加速度1/1
  下层电机控制/1("电机扭矩 ") -> Scope/1, Mux/1
  Add/1 -> S1/1, [station1]
  MATLAB Function/2(v) -> 前车速度/1, Derivative/1, Gain4/1, To Workspace6/1, [Vqian]
  Derivative/1 -> [ax1]
  [station1] -> Sum/1
  Subsystem3/1(AV_Eng) -> [AV_eng]
  Subsystem3/2(R_M_TC) -> [R_M_TC]
  Subsystem3/4(Vx) -> [Vx]
  Subsystem3/5(station2) -> [Station2]
  [Station2] -> Sum/2
  Subsystem3/3(Rgear_Tr) -> [Ig]
  Sum/1 -> 车距/1, [Distance]
  [Distance] -> Mux1/2, Subtract/1
  Multiport Switch/1 -> 下层电机控制/1(a_des 期望加速度), 液压制动控制/1(ades)  "期望加速度"
  [Vx] -> Gain3/1
  Gain3/1 -> 安全距离模型/1(Vx)
  Mux1/1 -> 期望距离 跟随情况/1
  mps-->km/h1/1 -> S5/2
  w/1 -> 加速度限制/1
  Clock/1 -> MATLAB Function/1(time)
  [ydesire] -> Scope1/2, To Workspace2/1  "期望距离m"
  [Vx] -> Scope1/1, To Workspace1/1  "后车速度km/h"
  [Distance] -> Scope1/3, To Workspace3/1  "实际距离m"
  [ax] -> Derivative1/1, Scope1/4, To Workspace/1  "加速度m/s^2"
  Derivative1/1 -> Scope1/5, To Workspace4/1  "冲击度m/s^3"
  [soc] -> Scope1/6, To Workspace5/1  "燃油消耗：g"
  Gain4/1 -> Integrator/1
  Integrator/1 -> Add/2
  MATLAB Function/1(s0) -> Add/1
  Constant1/1 -> MATLAB Function/2(kaiguan)
  [Vx] -> PID2/2(Vreal)
  [vset] -> ACC-CC切换/1(vset)
  [Vqian] -> ACC-CC切换/2(vp)
  [Distance] -> ACC-CC切换/4(d)
  [ydesire] -> ACC-CC切换/5(d_des)
  [Vx] -> ACC-CC切换/3(v)
  Memory25/1 -> ACC-CC切换/6(lastmodel)
  ACC-CC切换/1(d_logic1) -> [d_logic1]
  ACC-CC切换/2(d_logic2) -> [d_logic2]
  [d_logic1] -> Scope2/1, To Workspace7/1
  [d_logic2] -> Scope2/2, To Workspace8/1
  [vset] -> To Workspace9/1
  [ACC_CC] -> Scope2/3, To Workspace10/1
  PID Controller1/1 -> Multiport Switch/2
  加速度限制/1 -> Multiport Switch/3, S4/1
  Mux3/1 -> Scope3/1
  [station1] -> Mux3/1  "Leading car dispalcement"
  [Station2] -> Mux3/2  "Ego car displacement"
  Mux4/1 -> Scope3/2
  [Vqian] -> Mux4/1  "Leading car speed"
  [Vx] -> Mux4/2  "Ego car speed"
  Mux5/1 -> Scope3/3
  [Distance] -> Mux5/1  "Inter-car diantance"
  [ydesire] -> Mux5/2  "Desired distance"
  [ACC_CC] -> ?  "Mode ACC==1"
  ACC-CC切换/3(u) -> [ACC_CC], Memory25/1
  Constant2/1 -> Multiport Switch/1
  [Station2] -> S2/1, 大于500m停止仿真/1
  大于500m停止仿真/1 -> Stop Simulation/1
  PNG策略/1(vset) -> PID1/1(Vset), S3/2, Memory/1  "vset"
  [Vx] -> S3/1, Saturation/1  "vreal"
  PNG策略/2(ID) -> [ID], Memory1/1, S3/3  "ID"
  Constant3/1 -> PNG策略/1(vbase)
  Constant4/1 -> PNG策略/2(ax)
  Memory/1 -> PNG策略/5(vset_last)
  Memory1/1 -> PNG策略/4(ID_last)
  PID2/1(ades) -> w/1
  Constant6/1 -> PNG策略/3(ax2)
  PID1/1(ades) -> w/2
  [Vx] -> PID1/2(Vreal)
  [mc_omega] -> Scope4/1  "rad/s"
  [Tm] -> Scope4/2  "N.M"
  [eff] -> Scope4/3  "eff"
  1-D Lookup Table/1 -> mps-->km/h1/1
  时间/1 -> 1-D Lookup Table/1
  [soc] -> Display/1, To Workspace11/1, S3/4
  Constant5/1 -> PID2/1(Vset)
  Saturation/1 -> S5/1

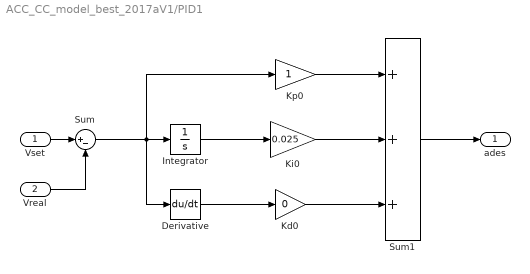
== system ACC_CC_model_best_2017aV1/PID1 ==
  Vset : Inport
  Vreal : Inport  Port=2
  Derivative : Derivative
  Integrator : Integrator
  Kd0 : Gain  Gain=0
  Ki0 : Gain  Gain=0.025
  Kp0 : Gain
  Sum : Sum  Inputs=|+-
  Sum1 : Sum  Inputs=+++
  ades : Outport
  wires:
  Vreal/1 -> Sum/2
  Sum/1 -> Kp0/1, Integrator/1, Derivative/1
  Derivative/1 -> Kd0/1
  Integrator/1 -> Ki0/1
  Vset/1 -> Sum/1
  Ki0/1 -> Sum1/2
  Kp0/1 -> Sum1/1
  Kd0/1 -> Sum1/3
  Sum1/1 -> ades/1

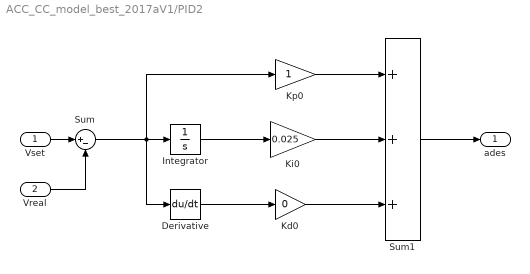
== system ACC_CC_model_best_2017aV1/PID2 ==
  Vset : Inport
  Vreal : Inport  Port=2
  Derivative : Derivative
  Integrator : Integrator
  Kd0 : Gain  Gain=0
  Ki0 : Gain  Gain=0.025
  Kp0 : Gain
  Sum : Sum  Inputs=|+-
  Sum1 : Sum  Inputs=+++
  ades : Outport
  wires:
  Sum1/1 -> ades/1
  Kd0/1 -> Sum1/3
  Kp0/1 -> Sum1/1
  Ki0/1 -> Sum1/2
  Vset/1 -> Sum/1
  Integrator/1 -> Ki0/1
  Derivative/1 -> Kd0/1
  Sum/1 -> Derivative/1, Integrator/1, Kp0/1
  Vreal/1 -> Sum/2

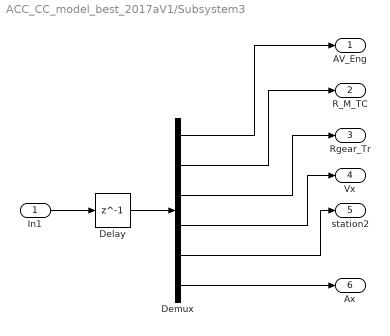
== system ACC_CC_model_best_2017aV1/Subsystem3 ==
  In1 : Inport
  Delay : Delay  DelayLength=1  InitialCondition=0
  Demux : Demux  Outputs=6
  AV_Eng : Outport
  R_M_TC : Outport  Port=2
  Rgear_Tr : Outport  Port=3
  Vx : Outport  Port=4
  station2 : Outport  Port=5
  Ax : Outport  Port=6
  wires:
  Demux/5 -> station2/1
  Demux/4 -> Vx/1
  Demux/3 -> Rgear_Tr/1
  Demux/2 -> R_M_TC/1
  Demux/1 -> AV_Eng/1
  In1/1 -> Delay/1
  Delay/1 -> Demux/1
  Demux/6 -> Ax/1

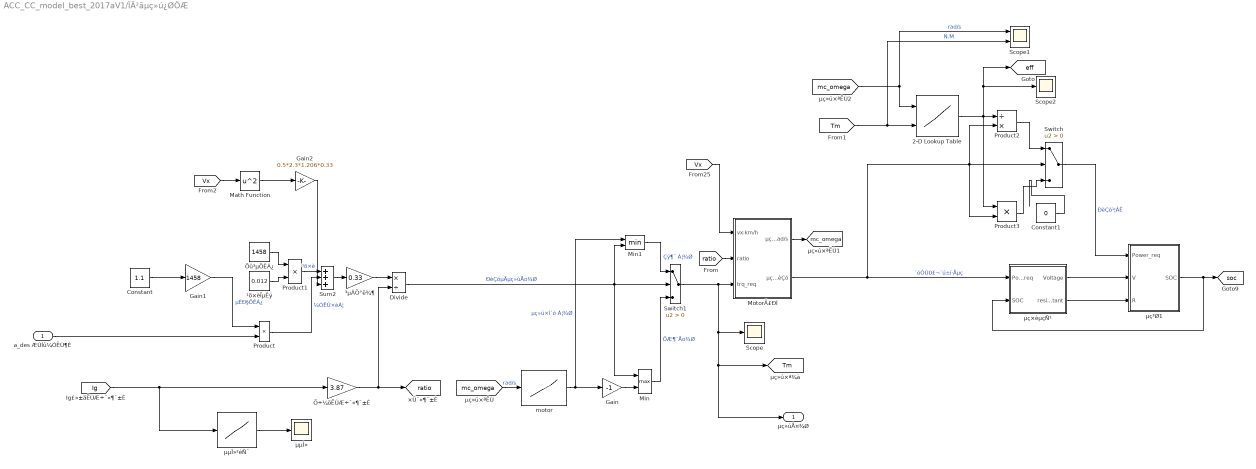
== system ACC_CC_model_best_2017aV1/下层电机控制 ==
  a_des 期望加速度 : Inport
  2-D Lookup Table : Lookup_n-D  BreakpointsForDimension1=mc_map_spd  BreakpointsForDimension2=mc_map_trq  Table=mc_eff_map  InternalRulePriority=Speed  RndMeth=Simplest  InputSameDT=on
  Constant : Constant  Value=1.1
  Constant1 : Constant  Value=0
  Divide : Product  Inputs=*/
  Gain : Gain  Gain=-1
  Gain1 : Gain  Gain=1458
  Gain2 : Gain  Gain=0.5*2.3*1.206*0.33
  Math Function : Math  Operator=square  SaturateOnIntegerOverflow=on
  Min : MinMax  Function=max  Inputs=2
  Min1 : MinMax  Inputs=2
  Motor模型 : Subsystem
  Product : Product
  Product1 : Product
  Product2 : Product  Inputs=/*
  Product3 : Product
  Scope : Scope
  Scope1 : Scope  NumInputPorts=2
  Scope2 : Scope
  Sum2 : Sum  Inputs=+++
  Switch : Switch  Criteria=u2 > Threshold
  Switch1 : Switch  Criteria=u2 > Threshold
  motor : Lookup_n-D  NumberOfTableDimensions=1  BreakpointsForDimension1=mc_map_spd  Table=mc_max_trq  ExtrapMethod=Clip  UseLastTableValue=on  InternalRulePriority=Speed  OutDataTypeStr=Inherit: Inherit from 'Table data'  RndMeth=Simplest  InputSameDT=on
  主减速器传动比 : Gain  Gain=3.87
  整车质量 : Constant  Value=1458
  档位 : Scope
  档位查询 : Lookup_n-D  NumberOfTableDimensions=1  BreakpointsForDimension1="[0.69 0.93 1.29 1.93  3.62 ]"  Table=[5 4 3 2 1]  InterpMethod=Cubic spline  ExtrapMethod=Cubic spline  InternalRulePriority=Speed  RndMeth=Simplest  InputSameDT=on
  滚阻系数 : Constant  Value=0.012
  电池1 : Subsystem
  电阻电压 : Subsystem
  车轮半径 : Gain  Gain=0.33
  "电机扭矩 " : Outport
  tag scope: Tm=global, eff=global, mc_omega=global, ratio=global, soc=global
  wires:
  主减速器传动比/1 -> [ratio], Divide/2
  Sum2/1 -> 车轮半径/1
  车轮半径/1 -> Divide/1
  Divide/1 -> Min1/2, Min/1, Switch1/2  "需求的电机扭矩"
  [Ig] -> 档位查询/1, 主减速器传动比/1
  Constant/1 -> Gain1/1
  Gain1/1 -> Product/1  "等效质量"
  a_des 期望加速度/1 -> Product/2
  整车质量/1 -> Product1/1
  滚阻系数/1 -> Product1/2
  Product/1 -> Sum2/2  "加速阻力"
  Product1/1 -> Sum2/1  "滚阻"
  档位查询/1 -> 档位/1
  电池1/1(SOC) -> 电阻电压/2(SOC), [soc]
  motor/1 -> Min1/1, Gain/1  "电机最大 力矩"
  [mc_omega] -> motor/1  "rad/s"
  Motor模型/2(电机功率需求) -> Switch/2, Product3/2, Product2/2, 电阻电压/1(Power_req)  "大于0，代表放电"
  电阻电压/2(resistant) -> 电池1/3(R)
  电阻电压/1(Voltage) -> 电池1/2(V)
  Motor模型/1(电机转速rad/s) -> [mc_omega]
  Min1/1 -> Switch1/1  "驱动 力矩"
  Gain/1 -> Min/2
  Min/1 -> Switch1/3  "制动扭矩"
  Switch1/1 -> Scope/1, "电机扭矩 "/1, [Tm], Motor模型/3(trq_req)
  [Vx] -> Motor模型/1(vx:km/h)
  [ratio] -> Motor模型/2(ratio)
  Switch/1 -> 电池1/1(Power_req)  "需求功率"
  [mc_omega] -> 2-D Lookup Table/1, Scope1/1  "rad/s"
  [Tm] -> Scope1/2, 2-D Lookup Table/2  "N.M"
  2-D Lookup Table/1 -> [eff], Scope2/1, Product3/1, Product2/1
  Product2/1 -> Switch/1
  Product3/1 -> Switch/3
  [Vx] -> Math Function/1
  Math Function/1 -> Gain2/1
  Gain2/1 -> Sum2/3
  Constant1/1 -> ?

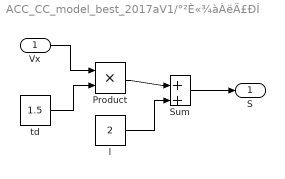
== system ACC_CC_model_best_2017aV1/安全距离模型 ==
  Vx : Inport
  Product : Product
  Sum : Sum  Inputs=+|+
  l : Constant  Value=2
  td : Constant  Value=1.5
  S : Outport
  wires:
  td/1 -> Product/2
  Vx/1 -> Product/1
  Product/1 -> Sum/1
  Sum/1 -> S/1
  l/1 -> Sum/2

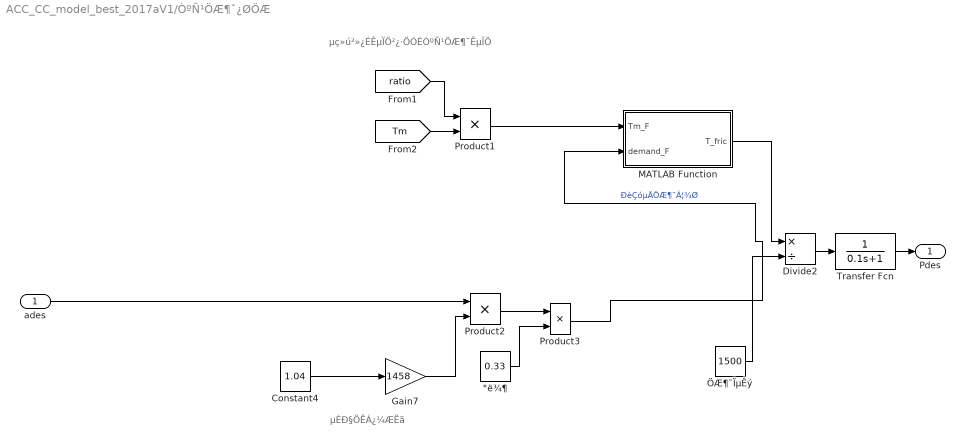
== system ACC_CC_model_best_2017aV1/液压制动控制 ==
  note: 电机不可实现部分由液压制动实现
  note: 等效质量计算
  ades : Inport
  Constant4 : Constant  Value=1.04
  Divide2 : Product  Inputs=*/
  Gain7 : Gain  Gain=1458
  MATLAB Function : MATLAB Function  TreatAsAtomicUnit=on
  Product1 : Product
  Product2 : Product
  Product3 : Product
  Transfer Fcn : TransferFcn  Denominator=[0.1 1]
  制动系数 : Constant  Value=1500
  半径 : Constant  Value=0.33
  "Pdes " : Outport
  wires:
  Constant4/1 -> Gain7/1
  Gain7/1 -> Product2/2
  Product2/1 -> Product3/1
  半径/1 -> Product3/2
  Product3/1 -> MATLAB Function/2(demand_F)  "需求的制动力矩"
  制动系数/1 -> Divide2/2
  Divide2/1 -> Transfer Fcn/1
  [Tm] -> Product1/2
  [ratio] -> Product1/1
  Product1/1 -> MATLAB Function/1(Tm_F)
  MATLAB Function/1(T_fric) -> Divide2/1
  ades/1 -> Product2/1
  Transfer Fcn/1 -> "Pdes "/1

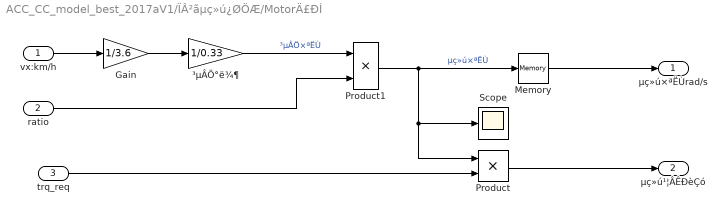
== system ACC_CC_model_best_2017aV1/下层电机控制/Motor模型 ==
  vx:km/h : Inport
  ratio : Inport  Port=2
  trq_req : Inport  Port=3
  Gain : Gain  Gain=1/3.6
  Memory : Memory  InheritSampleTime=on
  Product : Product  RndMeth=Zero
  Product1 : Product  RndMeth=Zero
  Scope : Scope
  车轮半径 : Gain  Gain=1/0.33
  电机转速rad/s : Outport
  电机功率需求 : Outport  Port=2
  wires:
  Product/1 -> 电机功率需求/1
  车轮半径/1 -> Product1/1  "车轮转速"
  ratio/1 -> Product1/2
  Product1/1 -> Product/1, Scope/1, Memory/1  "电机转速"
  Memory/1 -> 电机转速rad/s/1
  vx:km/h/1 -> Gain/1
  Gain/1 -> 车轮半径/1
  trq_req/1 -> Product/2

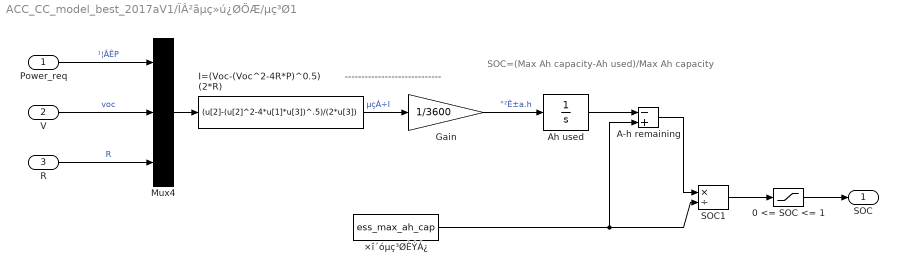
== system ACC_CC_model_best_2017aV1/下层电机控制/电池1 ==
  note: SOC=(Max Ah capacity-Ah used)/Max Ah capacity
  Power_req : Inport
  V : Inport  Port=2
  R : Inport  Port=3
  0 <= SOC <= 1 : Saturate  UpperLimit=1  LowerLimit=0
  A-h remaining : Sum  Inputs=-+  SaturateOnIntegerOverflow=on  InputSameDT=on  OutDataTypeStr=Inherit: Same as first input
  Ah used : Integrator  InitialCondition=(1-ess_init_soc)*ess_max_ah_cap
  Gain : Gain  Gain=1/3600
  I=(Voc-(Voc^2-4R*P)^0.5)        ----------------------------- (2*R) : Fcn  Expr=(u[2]-(u[2]^2-4*u[1]*u[3])^.5)/(2*u[3])
  Mux4 : Mux  Inputs=3
  SOC1 : Product  Inputs=*/  SaturateOnIntegerOverflow=on  RndMeth=Zero  InputSameDT=on  OutDataTypeStr=Inherit: Same as first input
  最大电池容量 : Constant  Value=ess_max_ah_cap
  SOC : Outport
  wires:
  I=(Voc-(Voc^2-4R*P)^0.5)        ----------------------------- (2*R)/1 -> Gain/1  "电流I"
  Ah used/1 -> A-h remaining/1
  Gain/1 -> Ah used/1  "安时a.h"
  A-h remaining/1 -> SOC1/1
  最大电池容量/1 -> SOC1/2, A-h remaining/2
  SOC1/1 -> 0 <= SOC <= 1/1
  V/1 -> Mux4/2  "voc"
  R/1 -> Mux4/3  "R"
  Mux4/1 -> I=(Voc-(Voc^2-4R*P)^0.5)        ----------------------------- (2*R)/1
  Power_req/1 -> Mux4/1  "功率P"
  0 <= SOC <= 1/1 -> SOC/1

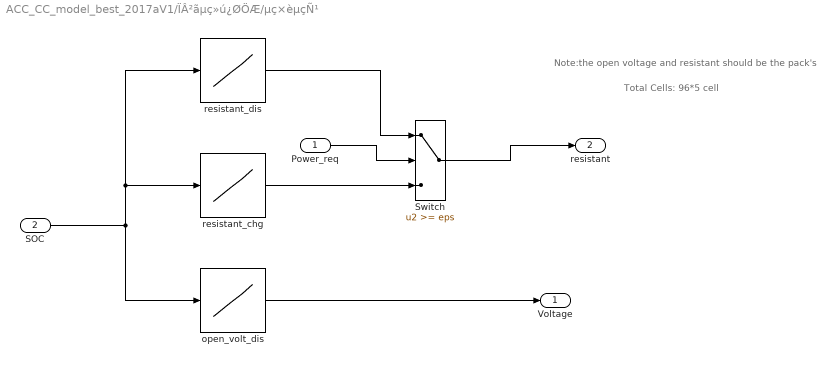
== system ACC_CC_model_best_2017aV1/下层电机控制/电阻电压 ==
  note: Note:the open voltage and resistant should be the pack's
  note: Total Cells: 96*5 cell
  Power_req : Inport
  SOC : Inport  Port=2
  Switch : Switch  Threshold=eps
  open_volt_dis : Lookup_n-D  NumberOfTableDimensions=1  BreakpointsForDimension1=ess_soc  Table=ess_voc  RndMeth=Simplest  InputSameDT=on
  resistant_chg : Lookup_n-D  NumberOfTableDimensions=1  BreakpointsForDimension1=ess_soc  Table=ess_r_chg  RndMeth=Simplest  InputSameDT=on
  resistant_dis : Lookup_n-D  NumberOfTableDimensions=1  BreakpointsForDimension1=ess_soc  Table=ess_r_dis  RndMeth=Simplest  InputSameDT=on
  Voltage : Outport
  resistant : Outport  Port=2
  wires:
  SOC/1 -> resistant_dis/1, resistant_chg/1, open_volt_dis/1
  open_volt_dis/1 -> Voltage/1
  Power_req/1 -> Switch/2
  Switch/1 -> resistant/1
  resistant_dis/1 -> Switch/1
  resistant_chg/1 -> Switch/3

== matlab function MATLAB Function ==
  data: s0 output double; time input double; kaiguan input double; v output double
function [s0,v] = fcn(time,kaiguan)
td=1.5;   %s;
% kaiguan=1~5代表ACC测试工况
% kaiguan=6~9代表ACC与CC切换控制策略测试工况

% 定速巡航遇到前车
% 前车换道离开I
% 前车换道离开II
% 前车加速离开


switch kaiguan
    
    case 1  %% ******************************************* 前车急加速工况1
        %前车急加速仿真工况 9s 内前车以 60km/h 匀速行驶，
        %本车以相同的速度与前车保持在27m 的距离跟随前车，
        %前车突然以 1.6m/s^2加速至90km/h .
        if time<30
            v=60;
        else
            v=60+1.6*(time-30)*3.6;  %以1.6m/s^2的加速度加速
            if v>90
                v=90;
            end
        end
        s0=60/3.6*td+2;%初始前车位置
    case 2  %% ******************************************* 前车急减速工况2
        % 在前 9s 内前车以 90km/h 的速度匀速行驶，
        % 本车以相同的速度与前车保持在 90/3.6*td+2 的距离跟随前车行驶，
        % 10s左右，以-1.6m/s2急减速至60km/h
        if time<9
            v=90;
        else
            v=90-1.6*(time-9)*3.6;  %以1.6m/s^2的加速度加速
            if v<60
                v=60;
            end
        end
        s0=90/3.6*td+2;%初始前车位置
    case 3  %% ******************************************* 稳态跟随工况3
        %前车以较小的加速度使车速不断在 90km/h 附近内波动
        % figure
        % x=0:0.001:50;
        % y=sin(x*0.1)+sin(x*0.4)-sin(x*0.2)+sin(x*0.8)-sin(x*0.3);
        % plot(x,y)
        x=time;
        v=sin(x*0.1)+sin(x*0.4)-sin(x*0.2)+sin(x*0.8)-sin(x*0.3)+90;
        s0=90/3.6*td+2;%初始前车位置
    case 4  %% ******************************************* 前车切入仿真工况 4：
        % 前15s内前车以80km/h 的速度匀速行驶，本车以相同
        % 的速度与前车保持在 45m 的距离跟随前车稳态行驶，
        % 在第15s 时，旁边车道车辆突然以 80km/h 的速度在本车前方 20m 处插入行车队列，
        % 导致本车与前车的实际距离远小于此速度下的期望的安全距离。
        if time<15
            s0=80/3.6*td+2;%初始前车位置
            v=80;
        else
            s0=80/3.6*td+2-15.3333;%初始前车位置(模拟切入一个车的情况)
            v=80;
        end
    case 5  %% ******************************************* 前车切出仿真工况 5：
        % 前 10s 内前车以 80km/h 的速度匀速行驶，本车以相同的速度与前车保持在 35m 的距离跟随前车行驶，在第 10s 时，前方车辆突然驶离
        % 本车道，而 ACC 系统传感器马上定位到前方同车道 70m 处速度同样为 80km/h 的另一车辆。
        if time<10
            v=80;
            s0=80/3.6*td+2;%初始前车位置
        else
            v=80;
            s0=80/3.6*td+2+35;%初始前车位置(模拟突然某车切出消失的情况)
        end
    case 6  %% ******************************************* 定速巡航遇到前车 1   ————————————ACC-CC切换策略
        %  本车以 80km/h 的速度做定速巡航运动，而前车以60km/h 的速度做匀速运动，本车与前车的初始距离为 200m，由于本车速度(巡航速度)
        % 大于前车速度，因此本车会在模式切换策略的控制下，在合适的时机由速度控制模式切换为距离控制模式，通过本工况可以检验模式切换策略
        % 由 CC 模式切换到 ACC 模式的切换时机的好坏
        v=60;
        s0=200;%初始前车位置
    case 7  %% ******************************************* 前车换道离开A   ————————————ACC-CC切换策略
        % 前车以 65km/h 的速度匀速行驶，本车同样以 65km/h的速度并与前车保持 35m 的距离跟随前车运动，在第 9s 时，前车突然换道离开，并
        % 且本车前方无行驶车辆，因此，本车由 ACC 模式切换到 CC 模式， CC 模式的巡航速度 80km/h。
        if time<9
            v=65;
            s0=v/3.6*td+2;%初始前车位置
        else
            v=0;
            s0=10000;%模拟前车换道消失
        end
        
    case 8  %% ******************************************* 前车换道离开B  ————————————ACC-CC切换策略
        % 前车以 100km/h 的速度匀速行驶，本车处于ACC 模式以相同的速度跟随前车行驶，在第 9s 时，前车换道离开，但本车前方
        % 80 处依然有汽车以 70km/h 的速度匀速行驶
        if time<9
            v=100;
            s0=v/3.6*td+2;%初始前车位置
        else
            v=70;
            s0=80;%模拟前车换道消失,前方80m处还有车辆70km/h前进
        end
        
    otherwise  %% ******************************************* 前车加速离开   ————————————ACC-CC切换策略
        % 前9s 内，前车以 60km/h
        % 的速度匀速行驶，本车相同速度跟车，9s时，前车以2.5m/s^2加速至90，然后以90km/h运输。本车的巡航车速为80km/h
        if time<9
            v=60;
        else
            v=60+2.5*(time-9)*3.6;  %以2.5m/s^2的加速度加速
            if v>90
                v=90;
            end
        end
        s0=60/3.6*td+2;%初始前车位置
end

== matlab function PNG策略 ==
  data: vset output double; vbase input double; ax input double; ax2 input double; ID_last input double; vset_last input double; ID output double
function [ vset,ID]    = fcn(vbase,ax, ax2,ID_last,vset_last)

if vset_last>vbase+5   %开始滑行
    ID=1;
    vset=vset_last+ax2*0.001;
    
elseif vset_last<vbase-5
    ID=0;
    vset=ax*0.001+vset_last;
else
    if ID_last>0  %上一时刻滑行
       ID=1;
       vset=vset_last+ax2*0.001;
    else
        ID=0;
        vset=vset_last+ax*0.001;
    end
end


end
